simulink model "gm_hdl_ofdm_tx"  (R2017b)
settings: Solver=FixedStepDiscrete  StartTime=0.0  StopTime=1  RelTol=1e-3
PreLoadFcn:
  | addpath('/home/mw/Documents/Design-Project/hdl_prj/hdlsrc/hdl_ofdm_tx');
libraries: commdigbbndam3 x16, hdlsllib x3, dspxfrm3 x1
CloseFcn:
  | addpath('/home/mw/Documents/Design-Project/hdl_prj/hdlsrc/hdl_ofdm_tx');
  | rmpath('/home/mw/Documents/Design-Project/hdl_prj/hdlsrc/hdl_ofdm_tx');
settings Model: Creator=jake  LastModifiedBy=mw
settings DataIOCC: SaveOutput=off  SaveTime=off
settings OptimizationCC: BlockReduction=off  ConditionallyExecuteInputs=off  DefaultParameterBehavior=Inlined
settings DebuggingCC: AlgebraicLoopMsg=error  InheritedTsInSrcMsg=none  SingleTaskRateTransMsg=error  StrictBusMsg=ErrorOnBusTreatedAsVector
settings HardwareCC: ProdBitPerPointer=32  ProdBitPerSizeT=32  ProdBitPerPtrDiffT=32  ProdLargestAtomicFloat=None  ProdIntDivRoundTo=Undefined  ProdEndianess=Unspecified  ProdWordSize=32  ProdHWDeviceType=ASIC/FPGA->ASIC/FPGA  ProdEqTarget=off
settings CodeAppCC: StateflowObjectComments=on
settings GRTTargetCC: TargetLangStandard=C89/C90 (ANSI)

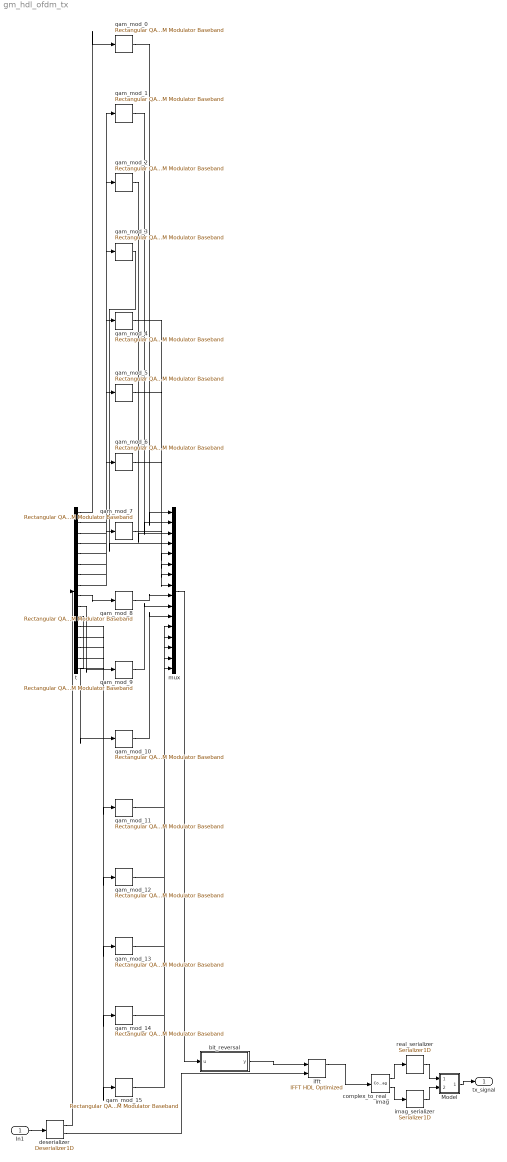
== system gm_hdl_ofdm_tx ==
  In1 : Inport  OutMin=0  OutMax=15  OutDataTypeStr=uint8  PortDimensions=[1]  SampleTime=0.0001
  Model : ModelReference  ModelNameDialog=gm_hdl_modulator  SimulationMode=Normal  ModelReferenceVersion=1.42
  bit_reversal : Subsystem
  complex_to_real_imag : ComplexToRealImag  SampleTime=0.0016
  deserializer : hdlsllib/HDL Operations/Deserializer1D  Ratio=16  IdleCycles=0  InitialCondition=fi(0,0,8,0,'hex','00')  startIn=off  validIn=off  validOut=on  inputDataDimensions=1  inputSampleTime=0.0001  inputSignalType=real
      settings: SourceProductName=HDL Coder  SourceProductBaseCode=HD
  ifft : dspxfrm3/IFFT HDL Optimized  FFTLength=16  Architecture=Streaming Radix 2^2  ComplexMultiplication=Use 3 multipliers and 5 adders  BitReversedOutput=off  BitReversedInput=on  Normalize=off  SimulateUsing=Code generation  RoundingMethod=Floor  ResetInputPort=off  StartOutputPort=off  EndOutputPort=off
      settings: SourceProductName=DSP System Toolbox  SourceProductBaseCode=DS
  imag_serializer : hdlsllib/HDL Operations/Serializer1D  Ratio=16  IdleCycles=0  validIn=off  startOut=off  validOut=off  inputDataDimensions=16  inputSampleTime=0.0016  inputSignalType=real
      settings: SourceProductName=HDL Coder  SourceProductBaseCode=HD
  mux : Mux  Inputs=16
  qam_mod_{0..15} (16 alike) : commdigbbndam3/Rectangular QAM Modulator Baseband  M=16  InType=Integer  Enc=Gray  Mapping=[0:15]  PowType=Min. distance between symbols  MinDist=2  AvgPow=1  PeakPow=1  Ph=0  outDtype=Fixed-point  outWordLen=16  outUDDataType=sfix(16)  outFracLenMode=Best precision  outFracLen=15  outDataTypeStr=fixdt(1,16)  outLastDataTypeStr=fixdt(1,16)
  real_serializer : hdlsllib/HDL Operations/Serializer1D  Ratio=16  IdleCycles=0  validIn=off  startOut=off  validOut=off  inputDataDimensions=16  inputSampleTime=0.0016  inputSignalType=real
      settings: SourceProductName=HDL Coder  SourceProductBaseCode=HD
  t : Demux  Outputs=16
  tx_signal : Outport
  wires:
  In1/1 -> deserializer/1
  Model/1 -> tx_signal/1
  mux/1 -> bit_reversal/1(u)
  bit_reversal/1(y) -> ifft/1
  complex_to_real_imag/1 -> real_serializer/1
  complex_to_real_imag/2 -> imag_serializer/1
  deserializer/1 -> t/1
  deserializer/2 -> ifft/2
  ifft/1 -> complex_to_real_imag/1
  imag_serializer/1 -> Model/2
  qam_mod_0/1 -> mux/1
  qam_mod_1/1 -> mux/2
  qam_mod_10/1 -> mux/11
  qam_mod_11/1 -> mux/12
  qam_mod_12/1 -> mux/13
  qam_mod_13/1 -> mux/14
  qam_mod_14/1 -> mux/15
  qam_mod_15/1 -> mux/16
  qam_mod_2/1 -> mux/3
  qam_mod_3/1 -> mux/4
  qam_mod_4/1 -> mux/5
  qam_mod_5/1 -> mux/6
  qam_mod_6/1 -> mux/7
  qam_mod_7/1 -> mux/8
  qam_mod_8/1 -> mux/9
  qam_mod_9/1 -> mux/10
  real_serializer/1 -> Model/1
  t/1 -> qam_mod_0/1
  t/2 -> qam_mod_1/1
  t/3 -> qam_mod_2/1
  t/4 -> qam_mod_3/1
  t/5 -> qam_mod_4/1
  t/6 -> qam_mod_5/1
  t/7 -> qam_mod_6/1
  t/8 -> qam_mod_7/1
  t/9 -> qam_mod_8/1
  t/10 -> qam_mod_9/1
  t/11 -> qam_mod_10/1
  t/12 -> qam_mod_11/1
  t/13 -> qam_mod_12/1
  t/14 -> qam_mod_13/1
  t/15 -> qam_mod_14/1
  t/16 -> qam_mod_15/1

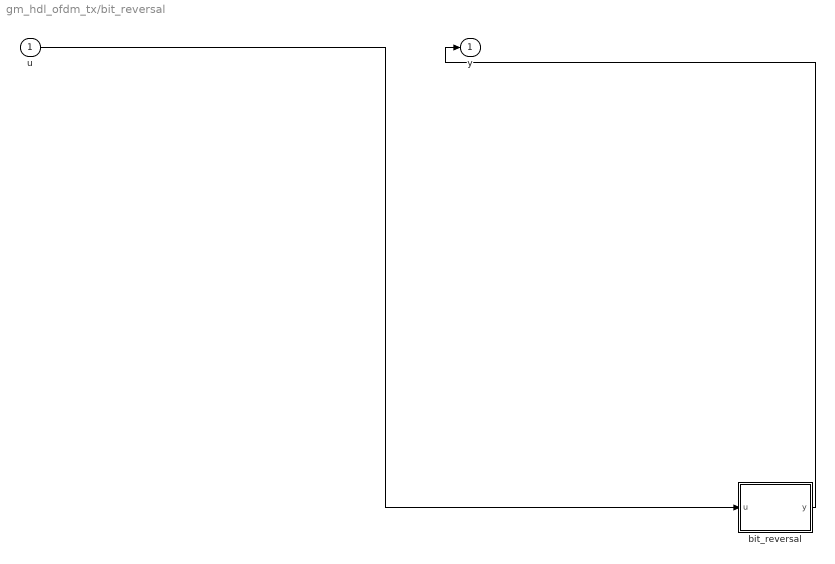
== system gm_hdl_ofdm_tx/bit_reversal ==
  u : Inport  PortDimensions=16  SampleTime=0.0016
  bit_reversal : MATLAB Function  TreatAsAtomicUnit=on
  y : Outport
  wires:
  u/1 -> bit_reversal/1(u)
  bit_reversal/1(y) -> y/1

== matlab function gm_hdl_ofdm_tx/bit_reversal/bit_reversal ==
  data: u input; y output
function y = bit_reverse(u)
    coder.varsize('bit-reverse', [1024 1]);
    u = bitrevorder(u);
    y = u;
end
